simulink model "Robot_Joint_Prototype11"  (R2018b)
settings: Solver=VariableStepAuto  StartTime=0.0  StopTime=4  RelTol=1e-3
values from neighbouring files (symbols this model uses):
  a = ( thf-thi )/( tb*( tf-tb ) )    [My_traj.m]    (also in Robot_Joint_Prarameter1.m = 0.244346095279; UR5_Mov.m = [a,ai(2:end)])
  b = b1    [My_traj.m]    (also in Robot_Joint_Prarameter1.m = 0)
  Dm = Dm1    [My_traj.m]    (also in Robot_Joint_Prarameter1.m = 1e-06)
  g = rgb2gray(J)    [Main.m]    (also in My_traj.m = g1; Robot_Joint_Prarameter1.m = 0)
  Jm = Jm1    [My_traj.m]    (also in Robot_Joint_Prarameter1.m = 1e-05)
  Ke = Ke1    [My_traj.m]    (also in Robot_Joint_Prarameter1.m = 0.05)
  l = l1    [My_traj.m]    (also in Robot_Joint_Prarameter1.m = 1)
  La = La1    [My_traj.m]    (also in Robot_Joint_Prarameter1.m = 0.0044)
  m = m1    [My_traj.m]    (also in Robot_Joint_Prarameter1.m = 1)
  N = N1    [My_traj.m]    (also in Robot_Joint_Prarameter1.m = 5)
  Ra = Ra1    [My_traj.m]    (also in Robot_Joint_Prarameter1.m = 10)
  tb = tb1    [My_traj.m]    (also in Robot_Joint_Prarameter1.m = 1; UR5_Mov.m = 1)
  thf = thf1*ToRad    [My_traj.m]    (also in Robot_Joint_Prarameter1.m = 1.74532925199)
  thi = thi1*ToRad    [My_traj.m]    (also in Robot_Joint_Prarameter1.m = 0.523598775598)
  ToDeg = 180/pi    (= 57.2957795131)    [My_fkine.m]    (also in My_traj.m; Robot_Joint_Prarameter1.m; UR5_Mdl.m; UR5_Mov.m)
  v = v1    [My_traj.m]    (also in Robot_Joint_Prarameter1.m = 10)
libraries: simulink x2
settings Model: Creator=Lnya  LastModifiedBy=Administrator
settings SolverCC: ZeroCrossAlgorithm=Adaptive
settings SFSimCC: SimUseLocalCustomCode=off
settings RTWCC: RTWUseLocalCustomCode=off
settings CodeAppCC: StateflowObjectComments=on

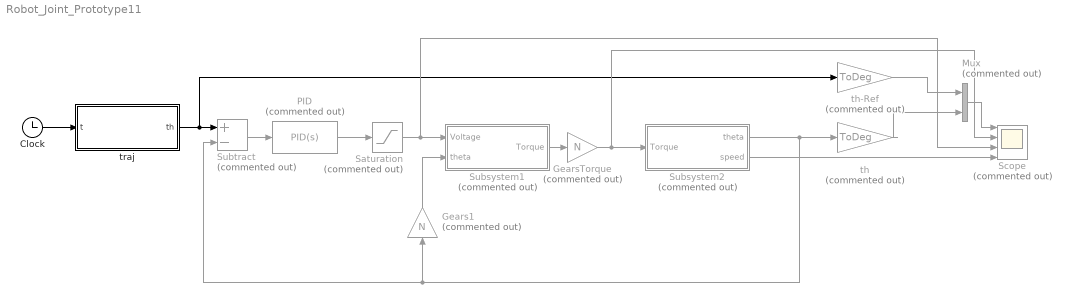
== system Robot_Joint_Prototype11 ==
  Clock : Clock
  Gears1 : Gain  Commented=on  Gain=N
  GearsTorque : Gain  Commented=on  Gain=N
  Mux : Mux  Commented=on  Inputs=2
  "PID " : simulink/Continuous/PID Controller  Commented=on  Controller=PID  Form=Parallel  TimeDomain=Continuous-time  SampleTime=-1  IntegratorMethod=Forward Euler  FilterMethod=Forward Euler  ControllerParametersSource=internal  P=1000  I=20  D=50  UseFilter=on  N=10  TunerSelectOption=Transfer Function Based (PID Tuner App)  InitialConditionSource=internal  InitialConditionForIntegrator=0  InitialConditionForFilter=0  DifferentiatorICPrevScaledInput=0  ExternalReset=none  TrackingMode=off  Kt=1  LimitOutput=off  UpperSaturationLimit=inf  LowerSaturationLimit=-inf  LinearizeAsGain=on  AntiWindupMode=none  Kb=1  POutMin=[]  POutMax=[]  IOutMin=[]  IOutMax=[]  DOutMin=[]  DOutMax=[]  NOutMin=[]  NOutMax=[]  SumOutMin=[]  SumOutMax=[]  SaturationOutMin=[]  SaturationOutMax=[]  PParamMin=[]  PParamMax=[]  IParamMin=[]  IParamMax=[]  DParamMin=[]  DParamMax=[]  NParamMin=[]  NParamMax=[]  KbParamMin=[]  KbParamMax=[]  KtParamMin=[]  KtParamMax=[]  KbOutMin=[]  KbOutMax=[]  KtOutMin=[]  KtOutMax=[]  IntegratorOutMin=[]  IntegratorOutMax=[]  FilterOutMin=[]  FilterOutMax=[]  SumI1OutMin=[]  SumI1OutMax=[]  SumI2OutMin=[]  SumI2OutMax=[]  SumI3OutMin=[]  SumI3OutMax=[]  SumI4OutMin=[]  SumI4OutMax=[]  SumDOutMin=[]  SumDOutMax=[]  DifferentiatorOutMin=[]  DifferentiatorOutMax=[]  FilterDiffOutCoefMin=[]  FilterDiffOutCoefMax=[]  ReciprocalOutMin=[]  ReciprocalOutMax=[]  SumDenOutMin=[]  SumDenOutMax=[]  SumNumOutMin=[]  SumNumOutMax=[]  DivideOutMin=[]  DivideOutMax=[]  IntegratorContinuousStateAttributes=''  IntegratorStateMustResolveToSignalObject=off  IntegratorRTWStateStorageClass=Auto  FilterContinuousStateAttributes=''  FilterStateMustResolveToSignalObject=off  FilterRTWStateStorageClass=Auto  ParallelPVariant=InternalParameters  IdealPVariant=Disabled  IVariant=InternalParameters  DVariant=InternalParameters  IntegratorVariant=Continuous  SatVariant=Disabled  AWVariant=Passthrough  PCopyVariant=Disabled  TRVariant=Disabled  FdbkBlocksVariant=Forward  IdealPFdbkVariant=Disabled  SatFdbkVariant=Disabled  DerivativeFilterVariant=ContFilter  NVariant=InternalParameters  NCopyVariant=Disabled  FilterICVariant=InternalICsFilter  IntegratorICVariant=InternalICs  ExternalResetVariant=Disabled  TRSumVariant=Passthrough  SumFdbkVariant=Disabled  SumVariant=Sum_PID
  Saturation : Saturate  Commented=on  UpperLimit=24  LowerLimit=-24
  Scope : Scope  Commented=on  NumInputPorts=4
  Subsystem1 : Subsystem  Commented=on
  Subsystem2 : Subsystem  Commented=on
  Subtract : Sum  Commented=on  Inputs=+-
  th : Gain  Commented=on  Gain=ToDeg
  th-Ref : Gain  Commented=on  Gain=ToDeg
  traj : Subsystem
  wires:
  Clock/1 -> traj/1(t)
  traj/1(th) -> th-Ref/1, Subtract/1
  Subtract/1 -> "PID "/1
  "PID "/1 -> Saturation/1
  Saturation/1 -> Subsystem1/1(Voltage), Scope/3
  Subsystem1/1(Torque) -> GearsTorque/1
  Gears1/1 -> Subsystem1/2(theta)
  GearsTorque/1 -> Scope/2, Subsystem2/1(Torque)
  th/1 -> Mux/2
  th-Ref/1 -> Mux/1
  Mux/1 -> Scope/1
  Subsystem2/2(speed) -> Scope/4
  Subsystem2/1(theta) -> Subtract/2, Gears1/1, th/1

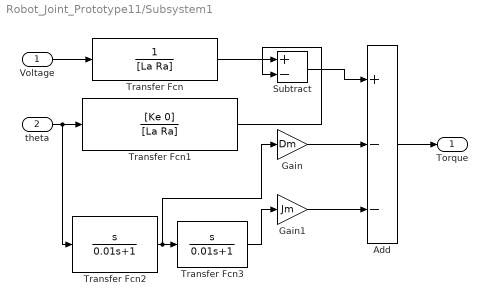
== system Robot_Joint_Prototype11/Subsystem1 ==
  Voltage : Inport
  theta : Inport  Port=2
  Add : Sum  Inputs=+--
  Gain : Gain  Gain=Dm
  Gain1 : Gain  Gain=Jm
  Subtract : Sum  Inputs=+-
  Transfer Fcn : TransferFcn  Denominator=[La Ra]
  Transfer Fcn1 : TransferFcn  Numerator=[Ke 0]  Denominator=[La Ra]
  Transfer Fcn2 : TransferFcn  Numerator=[1 0]  Denominator=[0.01 1]
  Transfer Fcn3 : TransferFcn  Numerator=[1 0]  Denominator=[0.01 1]
  Torque : Outport
  wires:
  Voltage/1 -> Transfer Fcn/1
  theta/1 -> Transfer Fcn2/1, Transfer Fcn1/1
  Transfer Fcn/1 -> Subtract/1
  Transfer Fcn1/1 -> Subtract/2
  Subtract/1 -> Add/1
  Gain/1 -> Add/2
  Gain1/1 -> Add/3
  Transfer Fcn2/1 -> Gain/1, Transfer Fcn3/1
  Transfer Fcn3/1 -> Gain1/1
  Add/1 -> Torque/1

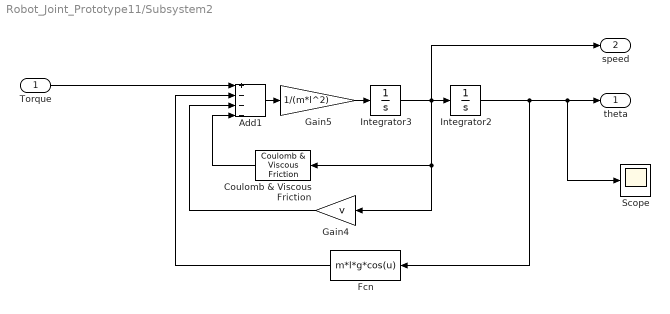
== system Robot_Joint_Prototype11/Subsystem2 ==
  Torque : Inport
  Add1 : Sum  Inputs=+---
  Coulomb & Viscous Friction : simulink/Discontinuities/Coulomb & Viscous Friction  offset=[b]  gain=0.00001
      settings: SourceProductName=Simulink
  Fcn : Fcn  Expr=m*l*g*cos(u)
  Gain4 : Gain  Gain=v
  Gain5 : Gain  Gain=1/(m*l^2)
  Integrator2 : Integrator  InitialCondition=thi
  Integrator3 : Integrator
  Scope : Scope
  theta : Outport
  speed : Outport  Port=2
  wires:
  Integrator3/1 -> speed/1, Coulomb & Viscous Friction/1, Gain4/1, Integrator2/1
  Integrator2/1 -> Scope/1, theta/1, Fcn/1
  Gain4/1 -> Add1/3
  Fcn/1 -> Add1/2
  Add1/1 -> Gain5/1
  Gain5/1 -> Integrator3/1
  Torque/1 -> Add1/1
  Coulomb & Viscous Friction/1 -> Add1/4

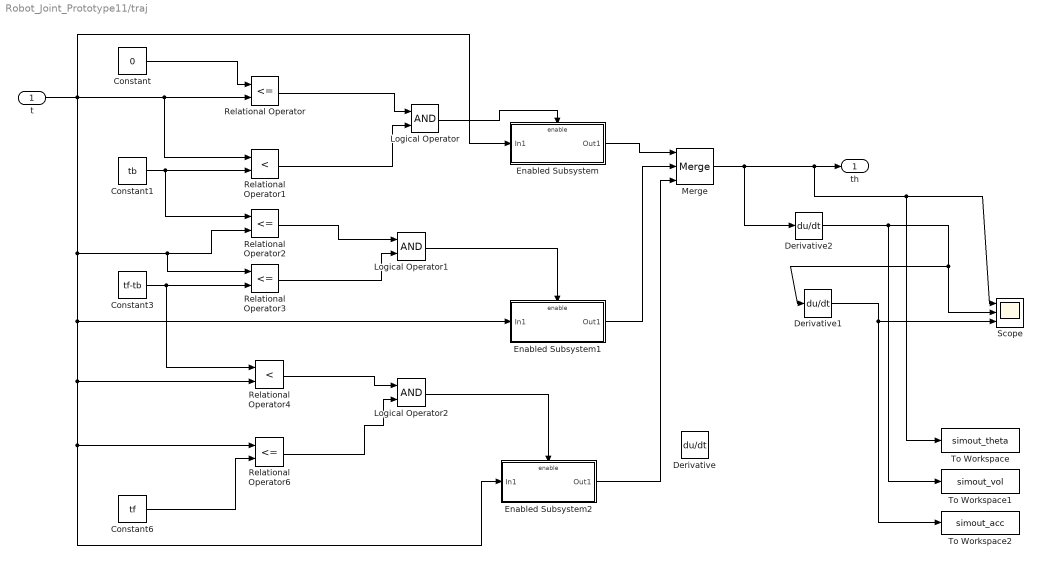
== system Robot_Joint_Prototype11/traj ==
  t : Inport
  Constant : Constant  Value=0
  Constant1 : Constant  Value=tb
  Constant3 : Constant  Value=tf-tb
  Constant6 : Constant  Value=tf
  Derivative : Derivative
  Derivative1 : Derivative
  Derivative2 : Derivative
  Enabled Subsystem : Subsystem  TreatAsAtomicUnit=on
  Enabled Subsystem1 : Subsystem  TreatAsAtomicUnit=on
  Enabled Subsystem2 : Subsystem  TreatAsAtomicUnit=on
  Logical Operator : Logic  AllPortsSameDT=off  OutDataTypeStr=boolean
  Logical Operator1 : Logic  AllPortsSameDT=off  OutDataTypeStr=boolean
  Logical Operator2 : Logic  AllPortsSameDT=off  OutDataTypeStr=boolean
  Merge : Merge  Inputs=3
  Relational Operator{,2..3,6} (4 alike) : RelationalOperator  Operator=<=  OutDataTypeStr=boolean  RndMeth=Simplest
  Relational Operator1 : RelationalOperator  Operator=<  OutDataTypeStr=boolean  RndMeth=Simplest
  Relational Operator4 : RelationalOperator  Operator=<  OutDataTypeStr=boolean  RndMeth=Simplest
  Scope : Scope  NumInputPorts=3
  To Workspace : ToWorkspace  VariableName=simout_theta  SampleTime=0.1
  To Workspace1 : ToWorkspace  VariableName=simout_vol  SampleTime=0.1
  To Workspace2 : ToWorkspace  VariableName=simout_acc  SampleTime=0.1
  th : Outport
  wires:
  Enabled Subsystem/1(Out1) -> Merge/1
  Enabled Subsystem1/1(Out1) -> Merge/2
  Enabled Subsystem2/1(Out1) -> Merge/3
  Constant/1 -> Relational Operator/1
  Relational Operator/1 -> Logical Operator/1
  Relational Operator1/1 -> Logical Operator/2
  Logical Operator/1 -> Enabled Subsystem/Enable
  Logical Operator1/1 -> Enabled Subsystem1/Enable
  Relational Operator3/1 -> Logical Operator1/2
  Relational Operator2/1 -> Logical Operator1/1
  Constant1/1 -> Relational Operator1/2, Relational Operator2/1
  Logical Operator2/1 -> Enabled Subsystem2/Enable
  Relational Operator6/1 -> Logical Operator2/2
  Relational Operator4/1 -> Logical Operator2/1
  t/1 -> Relational Operator2/2, Relational Operator3/1, Enabled Subsystem1/1(In1), Enabled Subsystem2/1(In1), Relational Operator6/1, Relational Operator4/2, Enabled Subsystem/1(In1), Relational Operator1/1, Relational Operator/2
  Constant6/1 -> Relational Operator6/2
  Constant3/1 -> Relational Operator3/2, Relational Operator4/1
  Merge/1 -> Derivative2/1, Scope/1, To Workspace/1, th/1
  Derivative2/1 -> To Workspace1/1, Derivative1/1, Scope/2
  Derivative1/1 -> Scope/3, To Workspace2/1

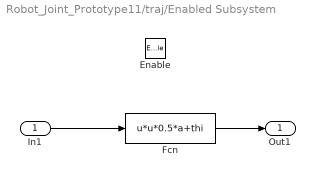
== system Robot_Joint_Prototype11/traj/Enabled Subsystem ==
  In1 : Inport
  Enable : EnablePort
  Fcn : Fcn  Expr=u*u*0.5*a+thi
  Out1 : Outport
  wires:
  In1/1 -> Fcn/1
  Fcn/1 -> Out1/1

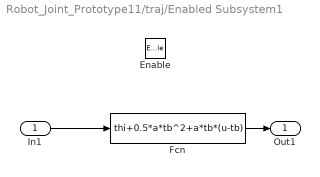
== system Robot_Joint_Prototype11/traj/Enabled Subsystem1 ==
  In1 : Inport
  Enable : EnablePort
  Fcn : Fcn  Expr=thi+0.5*a*tb^2+a*tb*(u-tb)
  Out1 : Outport
  wires:
  Fcn/1 -> Out1/1
  In1/1 -> Fcn/1

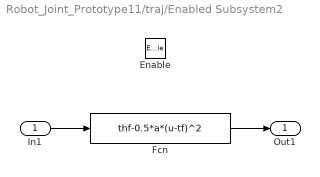
== system Robot_Joint_Prototype11/traj/Enabled Subsystem2 ==
  In1 : Inport
  Enable : EnablePort
  Fcn : Fcn  Expr=thf-0.5*a*(u-tf)^2
  Out1 : Outport
  wires:
  In1/1 -> Fcn/1
  Fcn/1 -> Out1/1
